simulink model "microchip_mcb_pmsm_foc_qep"  (R2021b)
settings: Solver=FixedStepDiscrete  StartTime=0.0  StopTime=8  FixedStep=Ts/2  RelTol=1e-3  EnableMultiTasking=on
InitFcn:
  | microchip_mcb_pmsm_foc_qep_data
values from neighbouring files (symbols this model uses):
  inverter = mcb_SetInverterParameters('Microchip_inverter')    [microchip_mcb_pmsm_foc_qep_data.m]
  PI_params = mcb.internal.SetControllerParameters(pmsm,inverter,PU_System,T_pwm,2*Ts,Ts_speed)    [microchip_mcb_pmsm_foc_qep_data.m]
  pmsm = mcb_SetPMSMMotorParameters('Microchip_motor')    [microchip_mcb_pmsm_foc_qep_data.m]
  PU_System = mcb_SetPUSystem(pmsm,inverter)    [microchip_mcb_pmsm_foc_qep_data.m]
  PWM_frequency = 20e3    (= 20000)    [microchip_mcb_pmsm_foc_qep_data.m]
  Ts = T_pwm    (= 5e-05)    [microchip_mcb_pmsm_foc_qep_data.m]
  Ts_motor = T_pwm/2    (= 2.5e-05)    [microchip_mcb_pmsm_foc_qep_data.m]
  Ts_simulink = T_pwm/2    (= 2.5e-05)    [microchip_mcb_pmsm_foc_qep_data.m]
  Ts_speed = 10*Ts    (= 0.0005)    [microchip_mcb_pmsm_foc_qep_data.m]
undefined symbols (not defined in the file or in its folder): A24, AD10, AD7, ADC0, LQFP144, MaxPer, ms, ns, PA0, PA1, PA10, PA11, PA12, PA13, PA18, PA9, PB0, PD18, PD19, PD24, PD25, PD26, Pin, Resol, SAME70Q21B, Unsigned, Vd_Ref_openLoop_PU
libraries: mcbcontrolslib x15, MCHP_Blockset x12, simulink x11, mcbpositiondecoderlib x4, mcbplantlib x1, autolibpmsmexterior x1
(part 4 of 4)

== system microchip_mcb_pmsm_foc_qep/Current Control/Closed Loop/OpenLoop/Mode Selector/If Action Subsystem2 ==
  Action Port : ActionPort  ActionPortLabel=else
  Constant : Constant  Value=0  OutDataTypeStr=dataType
  Constant1 : Constant  Value=0  OutDataTypeStr=Inherit: Inherit via back propagation
  Constant2 : Constant  OutDataTypeStr=Inherit: Inherit via back propagation
  Data Store Write : DataStoreWrite  DataStoreName=EnClosedLoop  IndexOptions=Index vector (dialog)  Indices=1  OutputSizes=1
  Data Store Write2 : DataStoreWrite  DataStoreName=EnPosOffset  IndexOptions=Index vector (dialog)  Indices=1  OutputSizes=1
  Out1 : Outport
  wires:
  Constant2/1 -> Data Store Write/1
  Constant1/1 -> Data Store Write2/1
  Constant/1 -> Out1/1

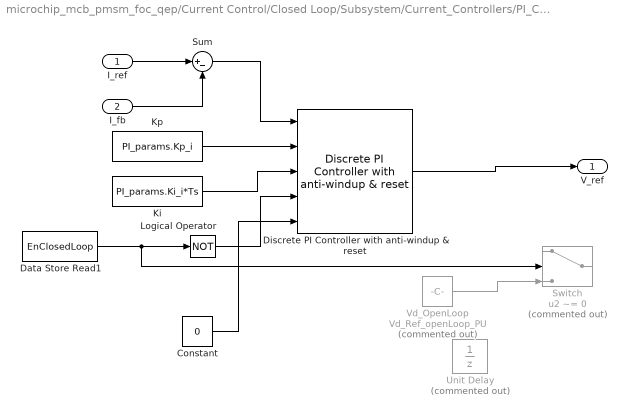
== system microchip_mcb_pmsm_foc_qep/Current Control/Closed Loop/Subsystem/Current_Controllers/PI_Controller_Id ==
  I_ref : Inport
  I_fb : Inport  Port=2
  Constant : Constant  Value=0  OutDataTypeStr=dataType
  Data Store Read1 : DataStoreRead  DataStoreName=EnClosedLoop  IndexOptions=Index vector (dialog)  Indices=1  OutputSizes=1
  Discrete PI Controller with anti-windup & reset : mcbcontrolslib/Discrete PI Controller  with anti-windup & reset  UpperSaturationLimit=1  LowerSaturationLimit=-1
      settings: SourceProductBaseCode=MT
  Ki : Constant  Value=PI_params.Ki_i*Ts  OutDataTypeStr=dataType  SampleTime=-1
  Kp : Constant  Value=PI_params.Kp_i  OutDataTypeStr=dataType  SampleTime=-1
  Logical Operator : Logic  Operator=NOT  IconShape=distinctive  AllPortsSameDT=off  OutDataTypeStr=boolean
  Sum : Sum  Inputs=|+-  OutDataTypeStr=Inherit: Same as first input
  Switch : Switch  Commented=on  Criteria=u2 ~= 0  RndMeth=Simplest
  Unit Delay : UnitDelay  Commented=on  SampleTime=-1  HasFrameUpgradeWarning=on
  Vd_OpenLoop : Constant  Commented=on  Value=Vd_Ref_openLoop_PU  OutDataTypeStr=dataType  SampleTime=-1
  V_ref : Outport  VectorParamsAs1DForOutWhenUnconnected=off
  wires:
  I_fb/1 -> Sum/2
  Sum/1 -> Discrete PI Controller with anti-windup & reset/1
  Kp/1 -> Discrete PI Controller with anti-windup & reset/2
  I_ref/1 -> Sum/1
  Ki/1 -> Discrete PI Controller with anti-windup & reset/3
  Logical Operator/1 -> Discrete PI Controller with anti-windup & reset/4
  Vd_OpenLoop/1 -> Switch/3
  Data Store Read1/1 -> Logical Operator/1, Switch/2
  Discrete PI Controller with anti-windup & reset/1 -> V_ref/1
  Constant/1 -> Discrete PI Controller with anti-windup & reset/5

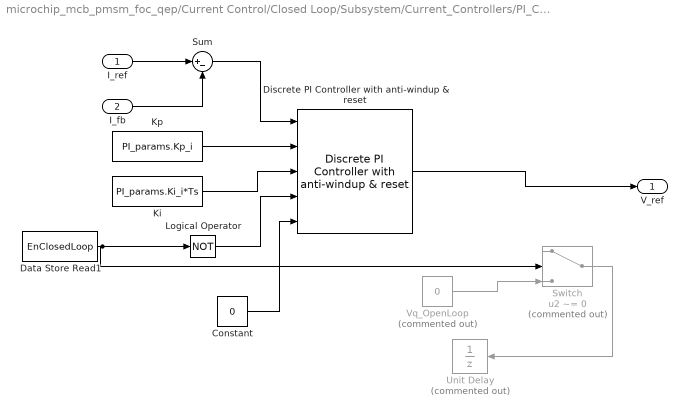
== system microchip_mcb_pmsm_foc_qep/Current Control/Closed Loop/Subsystem/Current_Controllers/PI_Controller_Iq ==
  I_ref : Inport
  I_fb : Inport  Port=2
  Constant : Constant  Value=0  OutDataTypeStr=dataType
  Data Store Read1 : DataStoreRead  DataStoreName=EnClosedLoop  IndexOptions=Index vector (dialog)  Indices=1  OutputSizes=1
  Discrete PI Controller with anti-windup & reset : mcbcontrolslib/Discrete PI Controller  with anti-windup & reset  UpperSaturationLimit=1  LowerSaturationLimit=-1
      settings: SourceProductBaseCode=MT
  Ki : Constant  Value=PI_params.Ki_i*Ts  OutDataTypeStr=dataType  SampleTime=-1
  Kp : Constant  Value=PI_params.Kp_i  OutDataTypeStr=dataType  SampleTime=-1
  Logical Operator : Logic  Operator=NOT  IconShape=distinctive  AllPortsSameDT=off  OutDataTypeStr=boolean
  Sum : Sum  Inputs=|+-  OutDataTypeStr=Inherit: Same as first input
  Switch : Switch  Commented=on  Criteria=u2 ~= 0  RndMeth=Simplest
  Unit Delay : UnitDelay  Commented=on  SampleTime=-1  HasFrameUpgradeWarning=on
  Vq_OpenLoop : Constant  Commented=on  Value=0  OutDataTypeStr=dataType  SampleTime=-1
  V_ref : Outport  VectorParamsAs1DForOutWhenUnconnected=off
  wires:
  Switch/1 -> Unit Delay/1
  I_fb/1 -> Sum/2
  Sum/1 -> Discrete PI Controller with anti-windup & reset/1
  Kp/1 -> Discrete PI Controller with anti-windup & reset/2
  I_ref/1 -> Sum/1
  Ki/1 -> Discrete PI Controller with anti-windup & reset/3
  Logical Operator/1 -> Discrete PI Controller with anti-windup & reset/4
  Vq_OpenLoop/1 -> Switch/3
  Data Store Read1/1 -> Switch/2, Logical Operator/1
  Constant/1 -> Discrete PI Controller with anti-windup & reset/5
  Discrete PI Controller with anti-windup & reset/1 -> V_ref/1

== system microchip_mcb_pmsm_foc_qep/Inverter and Motor - Plant Model/Plant Model/Inverter and Motor (sim)/Sensor_Measurements/Get_PU  ==
  rad : Inport
  Constant2 : Constant  Value=2*pi  OutDataTypeStr=single  SampleTime=-1
  Get_PU : Gain  Gain=1/(2*pi)  RndMeth=Simplest  OutDataTypeStr=Inherit: Same as input
  Mod : Math  Operator=mod  SaturateOnIntegerOverflow=on
  PU : Outport  VectorParamsAs1DForOutWhenUnconnected=off
  wires:
  rad/1 -> Mod/1
  Constant2/1 -> Mod/2
  Mod/1 -> Get_PU/1
  Get_PU/1 -> PU/1

== system microchip_mcb_pmsm_foc_qep/Inverter and Motor - Plant Model/Plant Model/Inverter and Motor (sim)/Sensor_Measurements/Wrap ==
  in : Inport
  Constant2 : Constant  OutDataTypeStr=single  SampleTime=-1
  Mod : Math  Operator=mod  SaturateOnIntegerOverflow=on
  out : Outport  VectorParamsAs1DForOutWhenUnconnected=off
  wires:
  in/1 -> Mod/1
  Constant2/1 -> Mod/2
  Mod/1 -> out/1
